simulink model "UAV_Simulation"  (R2021a)
settings: Solver=VariableStepAuto  StartTime=0.0  StopTime=180  RelTol=1e-3
values from neighbouring files (symbols this model uses):
  u1max = 12*pi/180    (= 0.209439510239)    [UAV_Initialization.m]
  u1min = -12*pi/180    (= -0.209439510239)    [UAV_Initialization.m]
  u2max = 25*pi/180    (= 0.436332312999)    [UAV_Initialization.m]
  u2min = -25*pi/180    (= -0.436332312999)    [UAV_Initialization.m]
  u3max = 5*pi/180    (= 0.0872664625997)    [UAV_Initialization.m]
  u3min = -5*pi/180    (= -0.0872664625997)    [UAV_Initialization.m]
  u4max = 1    [UAV_Initialization.m]
  x0 = [35 ... (first row only)    [UAV_Initialization.m]
undefined symbols (not defined in the file or in its folder): DCM, UAV_model_aerosonde
libraries: aerolibutil x2, aerolibfltsims x2, aerolibanimutils x1, vrlib x1
settings Model: Creator=Muhammad Owais Usman  LastModifiedBy=Muhammad Owais Usman

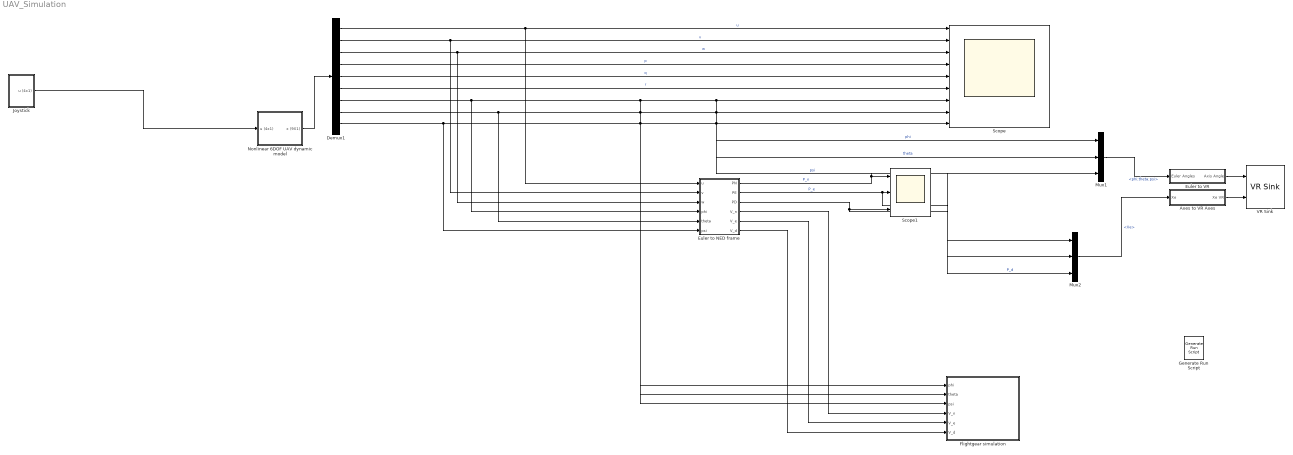
== system UAV_Simulation ==
  Axes to VR Axes : Subsystem
  Demux1 : Demux  Outputs=9
  Euler to NED frame : Subsystem
  Euler to VR : Subsystem
  Flightgear simulation : Subsystem
      mask Display: image('D:\Desktop\FlightGear_Logo_transparent.svg.png'); % Use "Edit Image" on toolstrip to change.
  Generate Run Script : aerolibfltsims/Generate Run Script  Architecture=Win64  dataFlow=Send  GeometryModelName=c172p  AirportId=PHNL  RunwayId=04L  InitialAltitude=7224  InitialHeading=113  OffsetDistance=4.72  OffsetAzimuth=0  InstallScenery=off  DisableShaders=on  OriginAddress=127.0.0.1  DestinationPort=5502  OriginPort=5505  LocalAddress=127.0.0.1  OutputFileName=runfg.bat  FlightGearBaseDirectory=C:\Program Files\FlightGear 2018.1.1
  Joystick : Subsystem
      mask Display: image('D:\Desktop\joystick.jpg'); % Use "Edit Image" on toolstrip to change.
  Mux1 : Mux  Inputs=3
  Mux2 : Mux  Inputs=3
  "Nonlinear 6DOF UAV dynamic model " : Subsystem
      mask Display: image('D:\Desktop\uav.jpg'); % Use "Edit Image" on toolstrip to change.
  Scope : Scope  NumInputPorts=9
  Scope1 : Scope  NumInputPorts=3
  VR Sink : vrlib/VR Sink  InstantiateOnLoad=on  SampleTime=0.1  ViewEnable=on  RemoteChange=off  RemoteView=off  FieldsWritten=HL20.rotation.4.1.1.double#HL20.translation.3.1.1.double  WorldFileName=aeroblk_HL20.wrl  WorldDescription=aeroblk_HL20  AutoView=on  VideoDimensions=[]  AllowVariableSize=off  FigureProperties="{'Position', 'Name', 'Viewpoint', 'CameraBound', 'CameraDirection', 'CameraPosition', 'CameraUpVector', 'ZoomFactor', 'Antialiasing', 'Headlight', 'Lighting', 'NavPanel', 'Sound', 'StatusBar', 'Stereo3D', 'Stereo3DCameraOffset', 'Stereo3DHIT', 'ToolBar', 'Textures', 'Transparency', 'Triad', 'Wireframe', 'NavZones', 'NavMode', 'NavSpeed', 'CaptureFileFormat', 'CaptureFileName', 'Record2DCompressMethod', 'Record2DCompressQuality', 'Record2D', 'Record2DFileName', 'Record2DFPS'; [5.0000000000000000e+00   9.2000000000000000e+01   5.7600000000000000e+02   3.5000000000000000e+02], 'aeroblk_HL20', 'Fixed Position', 'on', [0.0000000000000000e+00   0.0000000000000000e+00  -1.0000000000000000e+00], [0.0000000000000000e+00   0.0000000000000000e+00   0.0000000000000000e+00], [0.0000000000000000e+00   1.0000000000000000e+00   0.0000000000000000e+00], [1.0000000000000000e+00], 'on', 'on', 'on', 'halfbar', 'on', 'on', 'off', [1.0000000149011612e-01], [0.0000000000000000e+00], 'on', 'on', 'on', 'none', 'off', 'off', 'fly', 'normal', 'tif', '%f_anim_%n.tif', 'auto', [7.5000000000000000e+01], 'off', '%f_anim_%n.avi', 'auto'}"
  wires:
  "Nonlinear 6DOF UAV dynamic model "/1(x (9X1)) -> Demux1/1
  Demux1/6 -> Scope/6  "r"
  Demux1/5 -> Scope/5  "q"
  Demux1/4 -> Scope/4  "p"
  Demux1/3 -> Euler to NED frame/3(w), Scope/3  "w"
  Demux1/2 -> Euler to NED frame/2(v), Scope/2  "v"
  Demux1/1 -> Euler to NED frame/1(u), Scope/1  "u"
  Euler to VR/1(Axis Angle) -> VR Sink/1
  Mux2/1 -> Axes to VR Axes/1(Xe)  "<Xe>"
  Mux1/1 -> Euler to VR/1(Euler Angles)  "<phi;theta;psi>"
  Axes to VR Axes/1(Xe VR) -> VR Sink/2
  Demux1/7 -> Euler to NED frame/4(phi), Mux1/1, Scope/7, Flightgear simulation/1(phi)  "phi"
  Demux1/8 -> Euler to NED frame/5(theta), Mux1/2, Scope/8, Flightgear simulation/2(theta)  "theta"
  Demux1/9 -> Euler to NED frame/6(psi), Mux1/3, Scope/9, Flightgear simulation/3(psi)  "psi"
  Joystick/1(u (4x1)) -> "Nonlinear 6DOF UAV dynamic model "/1(u (4x1))
  Euler to NED frame/1(PN) -> Mux2/1, Scope1/1  "P_n"
  Euler to NED frame/3(PD) -> Mux2/3, Scope1/3  "P_d"
  Euler to NED frame/2(PE) -> Mux2/2, Scope1/2  "P_e"
  Euler to NED frame/4(V_n) -> Flightgear simulation/4(V_n)
  Euler to NED frame/5(V_e) -> Flightgear simulation/5(V_e)
  Euler to NED frame/6(V_d) -> Flightgear simulation/6(V_d)

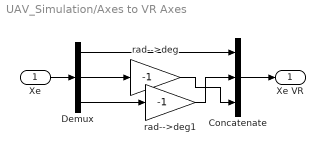
== system UAV_Simulation/Axes to VR Axes ==
  Xe : Inport
  Concatenate : Concatenate  NumInputs=3
  Demux : Demux  Outputs=3
      settings: DisplayOption=none
  rad-->deg : Gain  Gain=-1  SaturateOnIntegerOverflow=on  OutDataTypeStr=Inherit: Same as input  ParamDataTypeStr=Inherit: Same as input
  rad-->deg1 : Gain  Gain=-1  SaturateOnIntegerOverflow=on  OutDataTypeStr=Inherit: Same as input  ParamDataTypeStr=Inherit: Same as input
  Xe VR : Outport  VectorParamsAs1DForOutWhenUnconnected=off
  wires:
  Xe/1 -> Demux/1
  Demux/1 -> Concatenate/1
  Demux/2 -> rad-->deg/1
  Demux/3 -> rad-->deg1/1
  Concatenate/1 -> Xe VR/1
  rad-->deg1/1 -> Concatenate/2
  rad-->deg/1 -> Concatenate/3

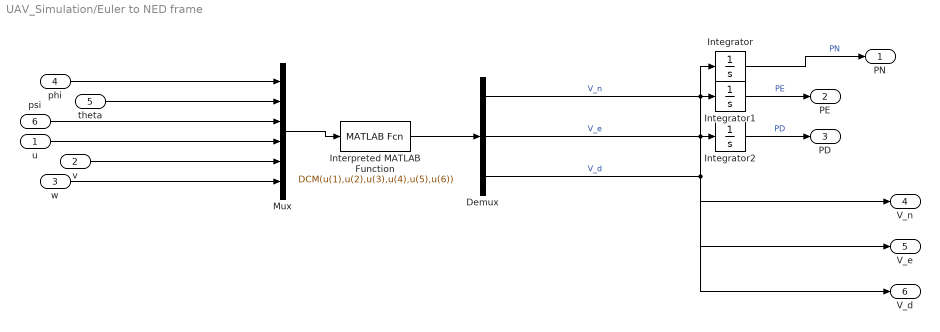
== system UAV_Simulation/Euler to NED frame ==
  u : Inport
  v : Inport  Port=2
  w : Inport  Port=3
  phi : Inport  Port=4
  theta : Inport  Port=5
  psi : Inport  Port=6
  Demux : Demux  Outputs=3
  Integrator : Integrator
  Integrator1 : Integrator
  Integrator2 : Integrator
  Interpreted MATLAB Function : MATLABFcn  MATLABFcn=DCM(u(1),u(2),u(3),u(4),u(5),u(6))  OutputDimensions=3  Output1D=off
  Mux : Mux  Inputs=6
  PN : Outport
  PE : Outport  Port=2
  PD : Outport  Port=3
  V_n : Outport  Port=4
  V_e : Outport  Port=5
  V_d : Outport  Port=6
  wires:
  Interpreted MATLAB Function/1 -> Demux/1
  Demux/3 -> Integrator2/1, V_d/1  "V_d"
  v/1 -> Mux/5
  Integrator2/1 -> PD/1  "PD"
  Mux/1 -> Interpreted MATLAB Function/1
  Demux/1 -> Integrator/1, V_n/1  "V_n"
  Demux/2 -> Integrator1/1, V_e/1  "V_e"
  Integrator1/1 -> PE/1  "PE"
  Integrator/1 -> PN/1  "PN"
  phi/1 -> Mux/1
  w/1 -> Mux/6
  theta/1 -> Mux/2
  psi/1 -> Mux/3
  u/1 -> Mux/4

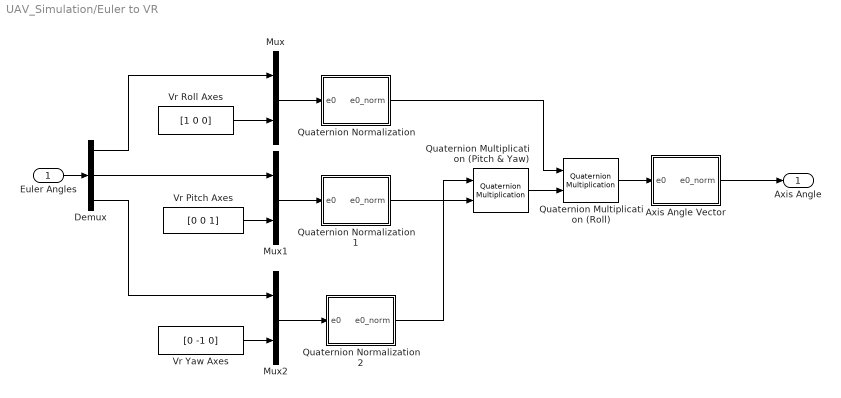
== system UAV_Simulation/Euler to VR ==
  Euler Angles : Inport
  Axis Angle Vector : Subsystem
  Demux : Demux  Outputs=3
      settings: DisplayOption=none
  Mux : Mux  Inputs=2
  Mux1 : Mux  Inputs=2
  Mux2 : Mux  Inputs=2
  Quaternion Multiplication (Pitch & Yaw) : aerolibutil/Quaternion Multiplication
  Quaternion Multiplication (Roll) : aerolibutil/Quaternion Multiplication
  Quaternion Normalization : Subsystem
  Quaternion Normalization1 : Subsystem
  Quaternion Normalization2 : Subsystem
  Vr Pitch Axes : Constant  Value=[0 0 1]
  Vr Roll Axes : Constant  Value=[1 0 0]
  Vr Yaw Axes : Constant  Value=[0 -1 0]
  Axis Angle : Outport  VectorParamsAs1DForOutWhenUnconnected=off
  wires:
  Quaternion Multiplication (Roll)/1 -> Axis Angle Vector/1(e0)
  Quaternion Multiplication (Pitch & Yaw)/1 -> Quaternion Multiplication (Roll)/2
  Axis Angle Vector/1(e0_norm) -> Axis Angle/1
  Quaternion Normalization/1(e0_norm) -> Quaternion Multiplication (Roll)/1
  Quaternion Normalization2/1(e0_norm) -> Quaternion Multiplication (Pitch & Yaw)/1
  Quaternion Normalization1/1(e0_norm) -> Quaternion Multiplication (Pitch & Yaw)/2
  Mux2/1 -> Quaternion Normalization2/1(e0)
  Mux1/1 -> Quaternion Normalization1/1(e0)
  Mux/1 -> Quaternion Normalization/1(e0)
  Demux/3 -> Mux2/1
  Vr Yaw Axes/1 -> Mux2/2
  Demux/2 -> Mux1/1
  Vr Pitch Axes/1 -> Mux1/2
  Demux/1 -> Mux/1
  Vr Roll Axes/1 -> Mux/2
  Euler Angles/1 -> Demux/1

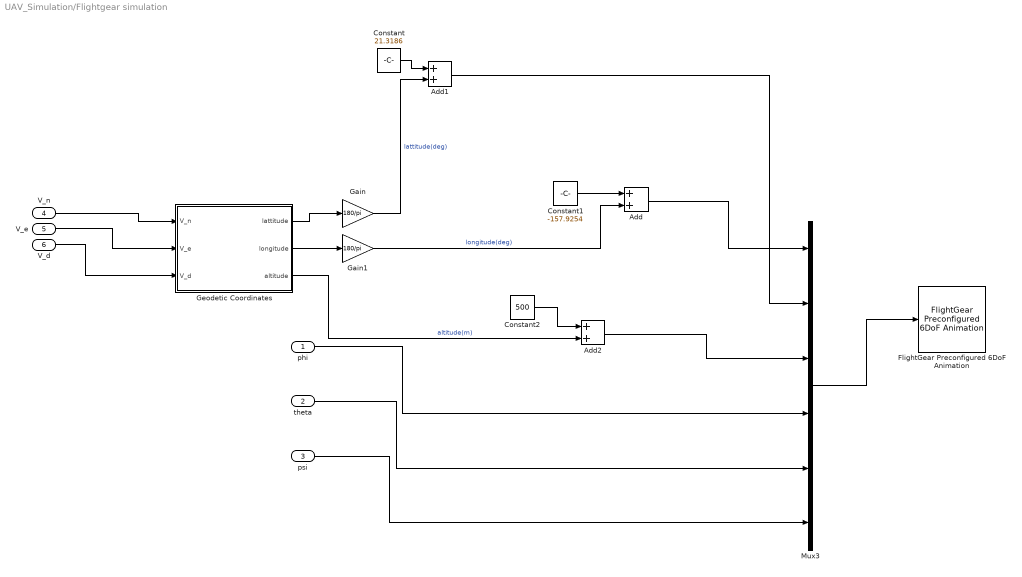
== system UAV_Simulation/Flightgear simulation ==
  phi : Inport
  theta : Inport  Port=2
  psi : Inport  Port=3
  V_n : Inport  Port=4
  V_e : Inport  Port=5
  V_d : Inport  Port=6
  Add : Sum
  Add1 : Sum
  Add2 : Sum
  Constant : Constant  Value=21.3186
  Constant1 : Constant  Value=-157.9254
  Constant2 : Constant  Value=500
  FlightGear Preconfigured 6DoF Animation : aerolibfltsims/FlightGear Preconfigured 6DoF Animation  xFlightGearVersion=v2019.1  DestinationIpAddress=127.0.0.1  DestinationPort=5502  SampleTime=1/30  packetVersion=24
  Gain : Gain  Gain=180/pi
  Gain1 : Gain  Gain=180/pi
  Geodetic Coordinates : Subsystem
  Mux3 : Mux  Inputs=6
  wires:
  psi/1 -> Mux3/6
  phi/1 -> Mux3/4
  Mux3/1 -> FlightGear Preconfigured 6DoF Animation/1
  Geodetic Coordinates/1(lattitude) -> Gain/1
  Geodetic Coordinates/2(longitude) -> Gain1/1
  theta/1 -> Mux3/5
  V_e/1 -> Geodetic Coordinates/2(V_e)
  V_n/1 -> Geodetic Coordinates/1(V_n)
  V_d/1 -> Geodetic Coordinates/3(V_d)
  Gain1/1 -> Add/2  "longitude(deg)"
  Constant1/1 -> Add/1
  Add/1 -> Mux3/1
  Gain/1 -> Add1/2  "lattitude(deg)"
  Constant/1 -> Add1/1
  Add1/1 -> Mux3/2
  Constant2/1 -> Add2/1
  Geodetic Coordinates/3(altitude) -> Add2/2  "altitude(m)"
  Add2/1 -> Mux3/3

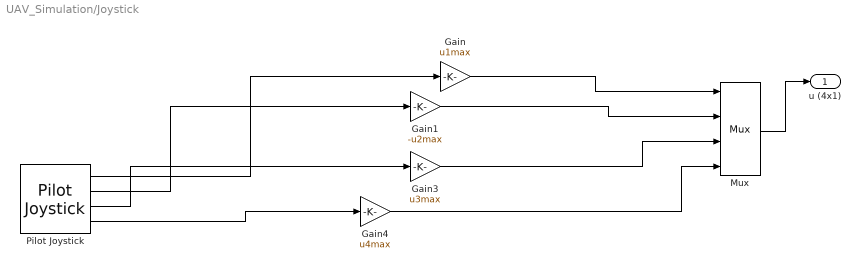
== system UAV_Simulation/Joystick ==
  Gain : Gain  Gain=u1max
  Gain1 : Gain  Gain=-u2max
  Gain3 : Gain  Gain=u3max
  Gain4 : Gain  Gain=u4max
  Mux : Mux
  Pilot Joystick : aerolibanimutils/Pilot Joystick  JoystickID=Joystick1  OutputConfiguration=FourAxis  SampleTime=1/30
  u (4x1) : Outport
  wires:
  Mux/1 -> u (4x1)/1
  Gain4/1 -> Mux/4
  Gain/1 -> Mux/1
  Gain3/1 -> Mux/3
  Gain1/1 -> Mux/2
  Pilot Joystick/1 -> Gain/1
  Pilot Joystick/2 -> Gain1/1
  Pilot Joystick/3 -> Gain3/1
  Pilot Joystick/4 -> Gain4/1

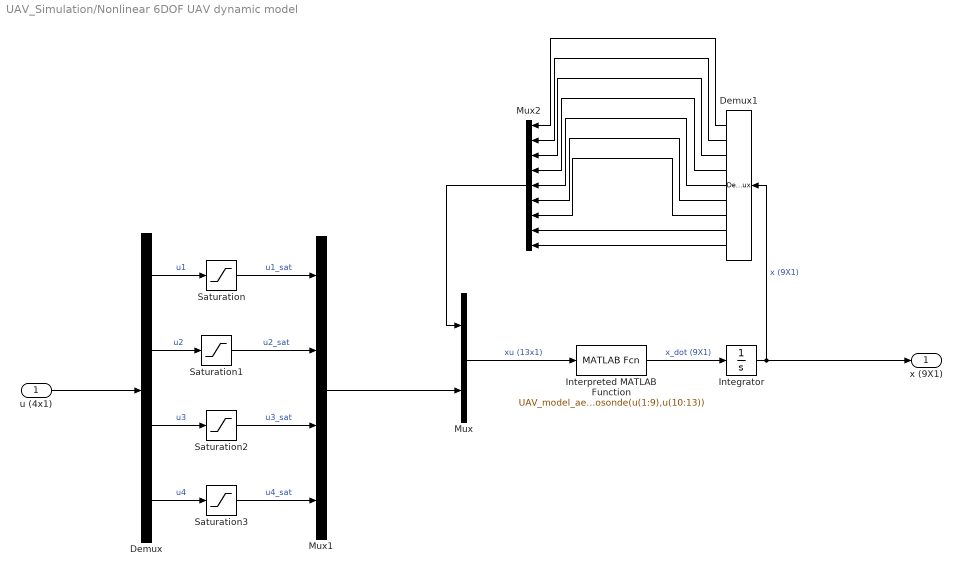
== system UAV_Simulation/Nonlinear 6DOF UAV dynamic model  ==
  u (4x1) : Inport
  Demux : Demux
  Demux1 : Demux  Outputs=9
  Integrator : Integrator  InitialCondition=x0
  Interpreted MATLAB Function : MATLABFcn  MATLABFcn=UAV_model_aerosonde(u(1:9),u(10:13))
  Mux : Mux  Inputs=2
  Mux1 : Mux
  Mux2 : Mux  Inputs=9
  Saturation : Saturate  UpperLimit=u1max  LowerLimit=u1min
  Saturation1 : Saturate  UpperLimit=u2max  LowerLimit=u2min
  Saturation2 : Saturate  UpperLimit=u3max  LowerLimit=u3min
  Saturation3 : Saturate  UpperLimit=u4max  LowerLimit=0
  x (9X1) : Outport
  wires:
  Mux/1 -> Interpreted MATLAB Function/1  "xu (13x1)"
  Integrator/1 -> Demux1/1, x (9X1)/1  "x (9X1)"
  Interpreted MATLAB Function/1 -> Integrator/1  "x_dot (9X1)"
  u (4x1)/1 -> Demux/1
  Demux/1 -> Saturation/1  "u1"
  Saturation/1 -> Mux1/1  "u1_sat"
  Demux/2 -> Saturation1/1  "u2"
  Demux/3 -> Saturation2/1  "u3"
  Demux/4 -> Saturation3/1  "u4"
  Saturation1/1 -> Mux1/2  "u2_sat"
  Saturation2/1 -> Mux1/3  "u3_sat"
  Saturation3/1 -> Mux1/4  "u4_sat"
  Mux1/1 -> Mux/2
  Mux2/1 -> Mux/1
  Demux1/9 -> Mux2/9
  Demux1/7 -> Mux2/7
  Demux1/6 -> Mux2/6
  Demux1/5 -> Mux2/5
  Demux1/4 -> Mux2/4
  Demux1/3 -> Mux2/3
  Demux1/2 -> Mux2/2
  Demux1/1 -> Mux2/1
  Demux1/8 -> Mux2/8

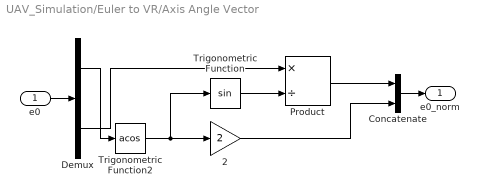
== system UAV_Simulation/Euler to VR/Axis Angle Vector ==
  e0 : Inport
  2 : Gain  Gain=2  SaturateOnIntegerOverflow=on  OutDataTypeStr=Inherit: Same as input  ParamDataTypeStr=Inherit: Same as input
  Concatenate : Concatenate
  Demux : Demux  Outputs=[1 3 ]
      settings: DisplayOption=none
  Product : Product  Inputs=*/  InputSameDT=on  SaturateOnIntegerOverflow=on  OutDataTypeStr=Inherit: Same as first input
  Trigonometric Function : Trigonometry
  Trigonometric Function2 : Trigonometry  Operator=acos
  e0_norm : Outport  VectorParamsAs1DForOutWhenUnconnected=off
  wires:
  Demux/1 -> Trigonometric Function2/1
  Demux/2 -> Product/1
  Concatenate/1 -> e0_norm/1
  Product/1 -> Concatenate/1
  2/1 -> Concatenate/2
  Trigonometric Function/1 -> Product/2
  Trigonometric Function2/1 -> Trigonometric Function/1, 2/1
  e0/1 -> Demux/1

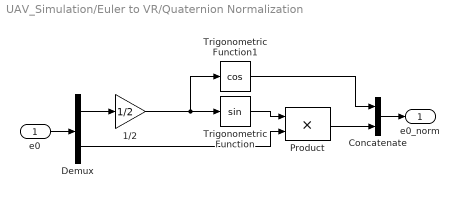
== system UAV_Simulation/Euler to VR/Quaternion Normalization ==
  e0 : Inport
  1/2 : Gain  Gain=1/2  SaturateOnIntegerOverflow=on  OutDataTypeStr=Inherit: Same as input  ParamDataTypeStr=Inherit: Same as input
  Concatenate : Concatenate
  Demux : Demux  Outputs=[1 3]
      settings: DisplayOption=none
  Product : Product  InputSameDT=on  SaturateOnIntegerOverflow=on  OutDataTypeStr=Inherit: Same as first input
  Trigonometric Function : Trigonometry
  Trigonometric Function1 : Trigonometry  Operator=cos
  e0_norm : Outport  VectorParamsAs1DForOutWhenUnconnected=off
  wires:
  Trigonometric Function1/1 -> Concatenate/1
  Demux/2 -> Product/2
  Demux/1 -> 1/2/1
  Concatenate/1 -> e0_norm/1
  Product/1 -> Concatenate/2
  Trigonometric Function/1 -> Product/1
  1/2/1 -> Trigonometric Function1/1, Trigonometric Function/1
  e0/1 -> Demux/1

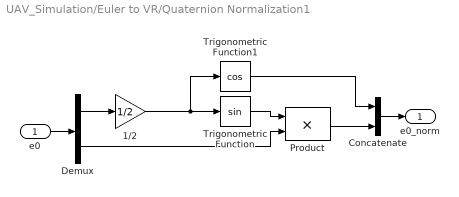
== system UAV_Simulation/Euler to VR/Quaternion Normalization1 ==
  e0 : Inport
  1/2 : Gain  Gain=1/2  SaturateOnIntegerOverflow=on  OutDataTypeStr=Inherit: Same as input  ParamDataTypeStr=Inherit: Same as input
  Concatenate : Concatenate
  Demux : Demux  Outputs=[1 3]
      settings: DisplayOption=none
  Product : Product  InputSameDT=on  SaturateOnIntegerOverflow=on  OutDataTypeStr=Inherit: Same as first input
  Trigonometric Function : Trigonometry
  Trigonometric Function1 : Trigonometry  Operator=cos
  e0_norm : Outport  VectorParamsAs1DForOutWhenUnconnected=off
  wires:
  e0/1 -> Demux/1
  1/2/1 -> Trigonometric Function/1, Trigonometric Function1/1
  Trigonometric Function/1 -> Product/1
  Product/1 -> Concatenate/2
  Concatenate/1 -> e0_norm/1
  Demux/1 -> 1/2/1
  Demux/2 -> Product/2
  Trigonometric Function1/1 -> Concatenate/1

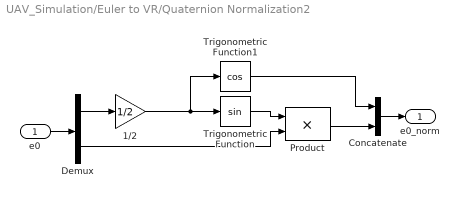
== system UAV_Simulation/Euler to VR/Quaternion Normalization2 ==
  e0 : Inport
  1/2 : Gain  Gain=1/2  SaturateOnIntegerOverflow=on  OutDataTypeStr=Inherit: Same as input  ParamDataTypeStr=Inherit: Same as input
  Concatenate : Concatenate
  Demux : Demux  Outputs=[1 3]
      settings: DisplayOption=none
  Product : Product  InputSameDT=on  SaturateOnIntegerOverflow=on  OutDataTypeStr=Inherit: Same as first input
  Trigonometric Function : Trigonometry
  Trigonometric Function1 : Trigonometry  Operator=cos
  e0_norm : Outport  VectorParamsAs1DForOutWhenUnconnected=off
  wires:
  Trigonometric Function1/1 -> Concatenate/1
  Demux/2 -> Product/2
  Demux/1 -> 1/2/1
  Concatenate/1 -> e0_norm/1
  Product/1 -> Concatenate/2
  Trigonometric Function/1 -> Product/1
  1/2/1 -> Trigonometric Function1/1, Trigonometric Function/1
  e0/1 -> Demux/1

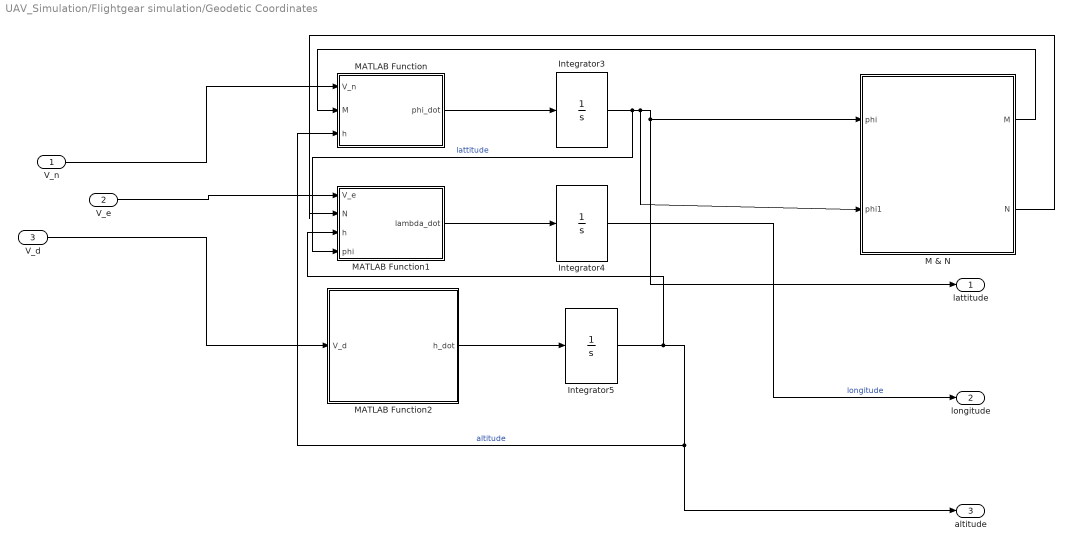
== system UAV_Simulation/Flightgear simulation/Geodetic Coordinates ==
  V_n : Inport
  V_e : Inport  Port=2
  V_d : Inport  Port=3
  Integrator3 : Integrator
  Integrator4 : Integrator
  Integrator5 : Integrator
  M & N : Subsystem
  MATLAB Function : MATLAB Function  TreatAsAtomicUnit=on
  MATLAB Function1 : MATLAB Function  TreatAsAtomicUnit=on
  MATLAB Function2 : MATLAB Function  TreatAsAtomicUnit=on
  lattitude : Outport
  longitude : Outport  Port=2
  altitude : Outport  Port=3
  wires:
  Integrator5/1 -> MATLAB Function1/3(h), altitude/1, MATLAB Function/3(h)  "altitude"
  M & N/1(M) -> MATLAB Function/2(M)
  Integrator3/1 -> MATLAB Function1/4(phi), M & N/2(phi1), lattitude/1, M & N/1(phi)  "lattitude"
  M & N/2(N) -> MATLAB Function1/2(N)
  MATLAB Function1/1(lambda_dot) -> Integrator4/1
  MATLAB Function/1(phi_dot) -> Integrator3/1
  V_e/1 -> MATLAB Function1/1(V_e)
  MATLAB Function2/1(h_dot) -> Integrator5/1
  Integrator4/1 -> longitude/1  "longitude"
  V_n/1 -> MATLAB Function/1(V_n)
  V_d/1 -> MATLAB Function2/1(V_d)

== system UAV_Simulation/Flightgear simulation/Geodetic Coordinates/M & N ==
  phi : Inport
  phi1 : Inport  Port=2
  MATLAB Function : MATLAB Function  TreatAsAtomicUnit=on
  MATLAB Function1 : MATLAB Function  TreatAsAtomicUnit=on
  M : Outport
  N : Outport  Port=2
  wires:
  phi/1 -> MATLAB Function/1(phi)
  phi1/1 -> MATLAB Function1/1(phi)
  MATLAB Function1/1(N) -> N/1
  MATLAB Function/1(M) -> M/1

== matlab function UAV_Simulation/Flightgear simulation/Geodetic Coordinates/M & N/MATLAB Function1 ==
  data: phi input; N output
function N = r_n(phi)

a = 6378137;
e = 0.081819190842622;

N = ( a )/ sqrt( 1 - (e^2)*(( sin(phi) )^2) );



end

== matlab function UAV_Simulation/Flightgear simulation/Geodetic Coordinates/M & N/MATLAB Function ==
  data: phi input; M output
function M = r_m(phi)
a = 6378137;
e = 0.081819190842622;

M = ( a*(1 - (e^2)) )/ (( 1 -(e^2)*( ((sin(phi))^2)) )^1.5);



end

== matlab function UAV_Simulation/Flightgear simulation/Geodetic Coordinates/MATLAB Function ==
  data: V_n input; M input; phi_dot output; h input
function phi_dot = latt_dot(V_n,M,h)

phi_dot = V_n/(M+h);


end

== matlab function UAV_Simulation/Flightgear simulation/Geodetic Coordinates/MATLAB Function1 ==
  data: V_e input; lambda_dot output; N input; h input; phi input
function lambda_dot = long_dot(V_e,N,h,phi)

lambda_dot = (V_e)/ ( (N+h)*cos(phi) );

end

== matlab function UAV_Simulation/Flightgear simulation/Geodetic Coordinates/MATLAB Function2 ==
  data: V_d input; h_dot output
function h_dot = altitude_dot(V_d)

h_dot = -V_d;


end
